simulink library "ControLibrary"  (R2015b)
settings: Solver=ode45  SolverMode=SingleTasking  StartTime=0.0  StopTime=10.0  RelTol=1e-3
values from neighbouring files (symbols this model uses):
  ControlSampleTime = 1/8000    (= 0.000125)    [initTPHardware.m]
  DCCC = initDCCC(LCL,SM)    [Sim_TP3_VSM_init.m]    (also in initDCCC.m = initHSS(LCL,SM))
undefined symbols (not defined in the file or in its folder): CCCTRL, DiscIntNeverNeededParam, VSMCTRL
undefined symbols (not defined in the file): HSS, VSMCC
libraries: FriedrichLibrary x46, simulink x23, simulink_extras x4, ControLibrary x2, ctrl_basic x2
(part 3 of 4)

== system ControLibrary/HSS/CONTROL/i_pi ==
  w : Inport
  x : Inport  Port=2
  umax : Inport  Port=3
  umin : Inport  Port=4
  x0 : Inport  Port=5
  Enable : EnablePort  StatesWhenEnabling=reset
  Discrete-Time Integrator : DiscreteIntegrator  InitialConditionSource=external  InitialConditionSetting=State (most efficient)  SampleTime=ControlSampleTime  ICPrevOutput=DiscIntNeverNeededParam  ICPrevScaledInput=DiscIntNeverNeededParam
  Sum : Sum  Inputs=|+-
  Sum1 : Sum  Inputs=|+-
  Sum2 : Sum  Inputs=++|
  Sum3 : Sum  Inputs=++|
  dynsat : simulink/Discontinuities/Saturation Dynamic  OutMin=[]  OutMax=[]  OutDataTypeStr=Inherit: Same as second input  OutDataType=fixdt(1, 16)  OutScaling=2^-10  DoSatur=off
  kaw : Gain  Gain=ki
  ki : Gain  Gain=ki
  kp : Gain  Gain=kp
  u : Outport
  wires:
  w/1 -> Sum/1
  x/1 -> Sum/2
  Sum/1 -> ki/1, kp/1
  Sum2/1 -> dynsat/2, Sum1/2
  dynsat/1 -> Sum1/1, u/1
  umin/1 -> dynsat/3
  umax/1 -> dynsat/1
  x0/1 -> Discrete-Time Integrator/2
  Discrete-Time Integrator/1 -> Sum2/1
  kp/1 -> Sum2/2
  ki/1 -> Sum3/2
  Sum3/1 -> Discrete-Time Integrator/1
  Sum1/1 -> kaw/1
  kaw/1 -> Sum3/1

== system ControLibrary/HSS/CONTROL/u_pi ==
  w : Inport
  x : Inport  Port=2
  umax : Inport  Port=3
  umin : Inport  Port=4
  x0 : Inport  Port=5
  Enable : EnablePort  StatesWhenEnabling=reset
  Discrete-Time Integrator : DiscreteIntegrator  InitialConditionSource=external  InitialConditionSetting=State (most efficient)  SampleTime=ControlSampleTime  ICPrevOutput=DiscIntNeverNeededParam  ICPrevScaledInput=DiscIntNeverNeededParam
  Sum : Sum  Inputs=|+-
  Sum1 : Sum  Inputs=|+-
  Sum2 : Sum  Inputs=++|
  Sum3 : Sum  Inputs=++|
  dynsat : simulink/Discontinuities/Saturation Dynamic  OutMin=[]  OutMax=[]  OutDataTypeStr=Inherit: Same as second input  OutDataType=fixdt(1, 16)  OutScaling=2^-10  DoSatur=off
  kaw : Gain  Gain=ki
  ki : Gain  Gain=ki
  kp : Gain  Gain=kp
  u : Outport
  wires:
  w/1 -> Sum/1
  x/1 -> Sum/2
  Sum/1 -> ki/1, kp/1
  Sum2/1 -> dynsat/2, Sum1/2
  dynsat/1 -> Sum1/1, u/1
  umin/1 -> dynsat/3
  umax/1 -> dynsat/1
  x0/1 -> Discrete-Time Integrator/2
  Discrete-Time Integrator/1 -> Sum2/1
  kp/1 -> Sum2/2
  ki/1 -> Sum3/2
  Sum3/1 -> Discrete-Time Integrator/1
  Sum1/1 -> kaw/1
  kaw/1 -> Sum3/1

== system ControLibrary/HSS/MANAGEMENT/RateLimit ==
  sp_DCBus : Inport
  ms_dcbus : Inport  Port=2
  Enable : EnablePort  StatesWhenEnabling=reset
  Abs : Abs
  Abs1 : Abs
  Add : Sum  Inputs=+-
  Add1 : Sum  Inputs=+-
  Compare To Constant1 : simulink/Logic and Bit Operations/Compare To Constant  relop=<  const=1  OutDataTypeStr=boolean
  Compare To Constant2 : simulink/Logic and Bit Operations/Compare To Constant  relop=<  const=10  OutDataTypeStr=boolean
  Constant : Constant  Value=UDCbusSpRateUp  SampleTime=ControlSampleTime
  Constant1 : Constant  Value=UDCbusSpRateDown  SampleTime=ControlSampleTime
  Ground : Ground
  Logical Operator : Logic  AllPortsSameDT=off  OutDataTypeStr=boolean
  S-R Flip-Flop : simulink_extras/Flip Flops/S-R Flip-Flop  initial_condition=0
  Saturation Dynamic : simulink/Discontinuities/Saturation Dynamic  OutMin=[]  OutMax=[]  OutDataTypeStr=Inherit: Same as second input  OutDataType=fixdt(1, 16)  OutScaling=2^-10  DoSatur=off
  Terminator : Terminator
  Vdc max : Constant  Value=UDCbusSpMax  SampleTime=ControlSampleTime
  Vdc min : Constant  Value=UDCbusSpMin  SampleTime=ControlSampleTime
  ratelimit1 : Subsystem  mask{Ts=ControlSampleTime}
      mask DialogControl ParameterGroupVar Prompt: Rate Limiter
  sp_DCBus_slow : Outport
  DCBus_isset : Outport  Port=2
  wires:
  ms_dcbus/1 -> ratelimit1/4(x0), Add1/2
  S-R Flip-Flop/1 -> DCBus_isset/1
  Ground/1 -> S-R Flip-Flop/2
  S-R Flip-Flop/2 -> Terminator/1
  Logical Operator/1 -> S-R Flip-Flop/1
  Compare To Constant2/1 -> Logical Operator/2
  Compare To Constant1/1 -> Logical Operator/1
  Abs1/1 -> Compare To Constant2/1
  Add1/1 -> Abs1/1
  Abs/1 -> Compare To Constant1/1
  Add/1 -> Abs/1
  Vdc max/1 -> Saturation Dynamic/1
  sp_DCBus/1 -> Saturation Dynamic/2
  Constant/1 -> ratelimit1/1(rateup)
  Constant1/1 -> ratelimit1/3(ratedown)
  Saturation Dynamic/1 -> ratelimit1/2(x), Add/2
  ratelimit1/1(x_slow) -> sp_DCBus_slow/1, Add/1, Add1/1
  Vdc min/1 -> Saturation Dynamic/3

== system ControLibrary/HSS/Meas/SI -> pu ==
  MeasIn : Inport
  Bus Creator1 : BusCreator  Inputs=5
  Bus Selector : BusSelector  OutputSignals=meas_u_out,meas_i_out,meas_i_inverter,meas_u_dc,meas_u_cap
  Normalize : Gain  Gain=1/PU.Ub  OutDataTypeStr=double  RndMeth=Round
  Normalize1 : Gain  Gain=1/PU.Ib  OutDataTypeStr=double  RndMeth=Round
  Normalize2 : Gain  Gain=1/PU.Ib  OutDataTypeStr=double  RndMeth=Round
  Normalize3 : Gain  Gain=1/PU.Ub  OutDataTypeStr=double  RndMeth=Round
  Normalize4 : Gain  Gain=1/PU.Ub/2  OutDataTypeStr=double  RndMeth=Round
  MeasOut : Outport
  wires:
  MeasIn/1 -> Bus Selector/1
  Normalize/1 -> Bus Creator1/1  "meas_u_out"
  Normalize1/1 -> Bus Creator1/3  "meas_i_inverter"
  Normalize2/1 -> Bus Creator1/2  "meas_i_out"
  Normalize4/1 -> Bus Creator1/4  "meas_vol_dc"
  Bus Creator1/1 -> MeasOut/1
  Bus Selector/1 -> Normalize/1  "<meas_u_out>"
  Bus Selector/2 -> Normalize2/1  "<meas_i_out>"
  Bus Selector/3 -> Normalize1/1  "<meas_i_inverter>"
  Bus Selector/4 -> Normalize4/1  "<meas_u_dc>"
  Bus Selector/5 -> Normalize3/1  "<meas_u_cap>"
  Normalize3/1 -> Bus Creator1/5  "meas_u_cap"

== system ControLibrary/VSM/CONTROL/VSMOC ==
  Manage : Inport
  Meas : Inport  Port=2
  u_inv_dq : Inport  Port=3
  Bus Selector1 : BusSelector  OutputSignals=enable_VSM.enable_ctrl,Param.VSM,enable_VSM.enable_inertia,sp_VSM
  Bus Selector11 : BusSelector  OutputSignals=phi
  Bus Selector2 : BusSelector  OutputSignals=PQ,PLL,u_cap.u_cap_dq0
  Selector : Selector  InputPortWidth=3  IndexOptions=Index vector (dialog)  Indices=[1 2]  OutputSizes=1
  Switch : Switch  Criteria=u2 ~= 0
  VSMOC : Subsystem
  phi_rad : Outport
  sp_u_inv_dq : Outport  Port=2  InitialOutput=[1 0]
  VSMdiag : Outport  Port=3
  wires:
  Selector/1 -> VSMOC/6(u_cap_dq0)
  Bus Selector2/3 -> Selector/1  "<u_cap_dq0>"
  u_inv_dq/1 -> VSMOC/7(u_inv_dq)
  Bus Selector1/4 -> VSMOC/3(sp_VSM)  "<sp_VSM>"
  Bus Selector1/3 -> VSMOC/2(enable_inertia)  "<enable_inertia>"
  Bus Selector1/2 -> VSMOC/1(Param)  "<VSM>"
  Bus Selector2/2 -> Bus Selector11/1, VSMOC/5(PLL)  "<PLL>"
  Bus Selector2/1 -> VSMOC/4(PQ_meas)  "<PQ>"
  Meas/1 -> Bus Selector2/1
  Bus Selector1/1 -> Switch/2, VSMOC/Enable  "<enable_ctrl>"
  Manage/1 -> Bus Selector1/1
  Switch/1 -> phi_rad/1
  VSMOC/2(sp_u_inv_dq) -> sp_u_inv_dq/1
  VSMOC/3(VSMdiag) -> VSMdiag/1
  VSMOC/1(phi_rad) -> Switch/1
  Bus Selector11/1 -> Switch/3  "<phi>"

== system ControLibrary/VSM/CONTROL/active_damping ==
  enable_damp_dq : Inport
  Reset : Inport  Port=2
  u_dq0 : Inport  Port=3
  Phi : Inport  Port=4
  Bus Selector : BusSelector  OutputSignals=Damp_dq,Damp_dq,Damp_CM,OmLead,OmLag
  Integrator (inertia) : DiscreteIntegrator  gainval=1  ExternalReset=rising  InitialConditionSource=external  InitialCondition=1  InitialConditionSetting=State (most efficient)  SampleTime=ControlSampleTime  ICPrevOutput=DiscIntNeverNeededParam  ICPrevScaledInput=DiscIntNeverNeededParam
  Mux : Mux  Inputs=3
  Product{,1..3} (4 alike) : Product
  Sum : Sum  Inputs=|+-
  Sum2 : Sum  Inputs=++|
  Unit Delay2 : UnitDelay  InitialCondition=[0 0 0]  SampleTime=ControlSampleTime
  dq0->ab0 phi : FriedrichLibrary/Transformations/dq0->ab0 phi  SystemSampleTime=-1
  damp_dq0 : Outport
  wires:
  Bus Selector/5 -> Product3/2  "<OmLag>"
  Bus Selector/4 -> Product2/1  "<OmLead>"
  dq0->ab0 phi/1 -> Integrator (inertia)/3
  Unit Delay2/1 -> dq0->ab0 phi/1
  Reset/1 -> Integrator (inertia)/2
  Phi/1 -> dq0->ab0 phi/2
  Product1/1 -> damp_dq0/1
  Mux/1 -> Product/1, Product1/1  "enable"
  Product/1 -> Product2/2, Sum2/1
  u_dq0/1 -> Product/2
  Bus Selector/3 -> Mux/3  "<Damp_CM>"
  Bus Selector/2 -> Mux/2  "<Damp_dq>"
  Bus Selector/1 -> Mux/1  "<Damp_dq>"
  enable_damp_dq/1 -> Bus Selector/1
  Sum/1 -> Integrator (inertia)/1
  Sum2/1 -> Product1/2, Product3/1
  Product3/1 -> Sum/2
  Integrator (inertia)/1 -> Sum2/2, Unit Delay2/1
  Product2/1 -> Sum/1

== system ControLibrary/VSM/CONTROL/dq0 to duty ==
  phi_rad : Inport
  u_dq0 : Inport  Port=2
  u_dc : Inport  Port=3
  Bias : Bias  Bias=Ctrl.PWM.tauT*Ctrl.PU.omegab
  Bus Creator3 : BusCreator  Inputs=2
  Divide : Product  Inputs=*/
  Gain : Gain  Gain=eye(NrChannels,3)  Multiplication=Matrix(K*u)
  Modulation : FriedrichLibrary/Transformations/Modulation  Method=Sine Modulation  Ts=ControlSampleTime
  Saturation : Saturate  UpperLimit=inf  LowerLimit=1
  Signal Specification1 : SignalSpecification
  dq0->ab0 phi : FriedrichLibrary/Transformations/dq0->ab0 phi  SystemSampleTime=-1
  d : Outport
  pwmDiag : Outport  Port=2
  wires:
  Signal Specification1/1 -> d/1
  Gain/1 -> Signal Specification1/1, Bus Creator3/1  "pwm"
  Bus Creator3/1 -> pwmDiag/1  "pwmDiag"
  Saturation/1 -> Divide/2
  u_dc/1 -> Saturation/1
  Bias/1 -> dq0->ab0 phi/2
  Modulation/1 -> Gain/1
  dq0->ab0 phi/1 -> Divide/1
  Divide/1 -> Modulation/1  "ab0 norm"
  u_dq0/1 -> dq0->ab0 phi/1
  phi_rad/1 -> Bias/1, Bus Creator3/2  "phi"

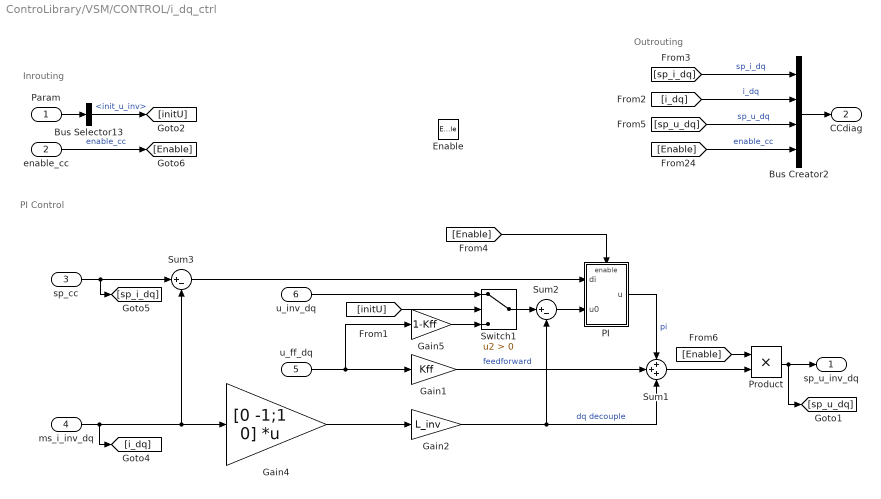
== system ControLibrary/VSM/CONTROL/i_dq_ctrl ==
  note: PI Control
  note: Outrouting
  note: Inrouting
  Param : Inport
  enable_cc : Inport  Port=2
  sp_cc : Inport  Port=3
  ms_i_inv_dq : Inport  Port=4
  u_ff_dq : Inport  Port=5
  u_inv_dq : Inport  Port=6
  Enable : EnablePort  StatesWhenEnabling=reset
  Bus Creator2 : BusCreator  Inputs=4
  Bus Selector13 : BusSelector  OutputSignals=init_u_inv
  Gain1 : Gain  Gain=Kff
  Gain2 : Gain  Gain=L_inv
  Gain4 : Gain  Gain=[0 -1;1 0]  Multiplication=Matrix(K*u)
  Gain5 : Gain  Gain=1-Kff
  PI : Subsystem
  Product : Product
  Sum1 : Sum  Inputs=+++
  Sum2 : Sum  Inputs=|+-
  Sum3 : Sum  Inputs=|+-
  Switch1 : Switch  Criteria=u2 > Threshold
  sp_u_inv_dq : Outport
  CCdiag : Outport  Port=2
  wires:
  Gain5/1 -> Switch1/3
  u_ff_dq/1 -> Gain5/1, Gain1/1
  [i_dq] -> Bus Creator2/2  "i_dq"
  [sp_i_dq] -> Bus Creator2/1  "sp_i_dq"
  Bus Creator2/1 -> CCdiag/1
  [Enable] -> Bus Creator2/4  "enable_cc"
  enable_cc/1 -> [Enable]  "enable_cc"
  [sp_u_dq] -> Bus Creator2/3  "sp_u_dq"
  Product/1 -> [sp_u_dq], sp_u_inv_dq/1
  [Enable] -> Product/1
  Bus Selector13/1 -> [initU]  "<init_u_inv>"
  Param/1 -> Bus Selector13/1
  sp_cc/1 -> [sp_i_dq], Sum3/1
  ms_i_inv_dq/1 -> Gain4/1, Sum3/2, [i_dq]
  Sum3/1 -> PI/1(di)
  [Enable] -> PI/Enable
  PI/1(u) -> Sum1/1  "pi"
  u_inv_dq/1 -> Switch1/1
  Sum1/1 -> Product/2
  [initU] -> Switch1/2
  Gain2/1 -> Sum2/2, Sum1/3  "dq decouple"
  Gain1/1 -> Sum1/2  "feedforward"
  Gain4/1 -> Gain2/1
  Sum2/1 -> PI/2(u0)
  Switch1/1 -> Sum2/1

== system ControLibrary/VSM/CONTROL/re_init ==
  Uset : Inport
  Uvr : Inport  Port=2
  Trigger : TriggerPort  PortDimensions=1
  MATLAB Function : MATLAB Function  TreatAsAtomicUnit=on
  Terminator : Terminator
  Uinit : Outport
  Phi : Outport  Port=2
  wires:
  MATLAB Function/2(Phi) -> Phi/1
  Uvr/1 -> MATLAB Function/2(Uvr)
  Uset/1 -> MATLAB Function/1(Uset)
  MATLAB Function/1(Uinit) -> Uinit/1
  MATLAB Function/3(UvrShift) -> Terminator/1

== system ControLibrary/VSM/MANAGEMENT/current_watchdog ==
  |i| set : Inport
  |i| reset : Inport  Port=2
  i_ab : Inport  Port=3
  sp_gain : Inport  Port=4
  active_current_watchdog : EnablePort  StatesWhenEnabling=reset
  Divide : Product  Inputs=/**
  Math Function1 : Math  Operator=square  SaturateOnIntegerOverflow=on
  Math Function2 : Math  Operator=square  SaturateOnIntegerOverflow=on
  Math Function3 : Math  Operator=square  SaturateOnIntegerOverflow=on
  Relational Operator : RelationalOperator  Operator=<=  OutDataTypeStr=boolean
  Relational Operator1 : RelationalOperator  Operator=<=  OutDataTypeStr=boolean
  S-R Flip-Flop1 : simulink_extras/Flip Flops/S-R Flip-Flop  initial_condition=0
  Sum of Elements1 : Sum  Inputs=+
  Terminator1 : Terminator
  enable_cc : Outport
  sp_gain_wd : Outport  Port=2
  wires:
  Divide/1 -> sp_gain_wd/1
  sp_gain/1 -> Divide/3
  |i| set/1 -> Math Function2/1, Divide/1
  |i| reset/1 -> Math Function3/1, Divide/2
  Math Function3/1 -> Relational Operator1/2
  S-R Flip-Flop1/1 -> enable_cc/1
  S-R Flip-Flop1/2 -> Terminator1/1
  Relational Operator/1 -> S-R Flip-Flop1/1
  Relational Operator1/1 -> S-R Flip-Flop1/2
  Math Function1/1 -> Sum of Elements1/1
  Sum of Elements1/1 -> Relational Operator/2, Relational Operator1/1
  i_ab/1 -> Math Function1/1
  Math Function2/1 -> Relational Operator/1

== system ControLibrary/VSM/MANAGEMENT/i_sp_dq_generator ==
  sp_gain : Inport
  i_dq : Inport  Port=2
  Trigger : TriggerPort  PortDimensions=1
  Gain : Gain  Commented=on  Gain=0.95/1.5
  Gain1 : Gain  Commented=on  Gain=eye(2,1)
  Gain3 : Gain  Commented=on  Gain=0.5
  Math Function : Math  Commented=on  Operator=square  SaturateOnIntegerOverflow=on
  Product : Product
  Saturation : Saturate  UpperLimit=1  LowerLimit=-1
  Saturation1 : Saturate  UpperLimit=1  LowerLimit=-1
  Sqrt : Sqrt  Commented=on  SaturateOnIntegerOverflow=on
  Sum of Elements : Sum  Commented=on  Inputs=+
  Terminator : Terminator  Commented=on
  Terminator1 : Terminator  Commented=on
  i_dq_spt : Outport
  wires:
  Saturation/1 -> Product/1
  sp_gain/1 -> Saturation/1
  Gain3/1 -> Terminator1/1
  Gain/1 -> Terminator/1
  i_dq/1 -> Product/2, Gain/1, Math Function/1
  Math Function/1 -> Sum of Elements/1
  Sum of Elements/1 -> Sqrt/1
  Sqrt/1 -> Gain1/1
  Gain1/1 -> Gain3/1
  Product/1 -> Saturation1/1
  Saturation1/1 -> i_dq_spt/1

== system ControLibrary/VSM/MANAGEMENT/sp_VSM ==
  EnableRateLimit : Inport
  CMD : Inport  Port=2
  MEAS : Inport  Port=3
  Bus Creator : BusCreator  Inputs=3
  Bus Selector1 : BusSelector  OutputSignals=u_out.u_out_ab0
  Bus Selector6 : BusSelector  OutputSignals=Param.VSM.sp_f,Param.VSM.sp_E,Param.VSM.sp_PQ,Param.VSM.sp_PQ_limit
  "CMD " : InportShadow  Port=2
  E(PQ) : Subsystem
  PQ(U) Limit : Subsystem
  RateLimit : Subsystem
  Saturation : Saturate  UpperLimit=1  LowerLimit=-1
  sp_VSM : Outport
  wires:
  Saturation/1 -> RateLimit/1(PQ)
  "CMD "/1 -> E(PQ)/2(cmd)
  Bus Creator/1 -> sp_VSM/1
  Bus Selector6/1 -> Bus Creator/1  "<sp_f>"
  MEAS/1 -> Bus Selector1/1
  CMD/1 -> Bus Selector6/1
  PQ(U) Limit/1(sp_PQ_limit) -> Bus Creator/3  "sp_PQ"
  Bus Selector6/4 -> PQ(U) Limit/2(enable)  "<sp_PQ_limit>"
  Bus Selector1/1 -> PQ(U) Limit/3(u_out)  "<u_out_ab0>"
  RateLimit/1(PQslow) -> PQ(U) Limit/1(sp_PQ), E(PQ)/3(sp_PQ)
  EnableRateLimit/1 -> RateLimit/Enable  "ENABLED"
  Bus Selector6/3 -> Saturation/1  "<sp_PQ>"
  Bus Selector6/2 -> E(PQ)/1(E)  "<sp_E>"
  E(PQ)/1(sp_E) -> Bus Creator/2  "sp_E"

== system ControLibrary/VSM/Meas/SI -> pu ==
  MeasIn : Inport
  Bus Creator1 : BusCreator  Inputs=5
  Bus Selector : BusSelector  OutputSignals=meas_u_out,meas_i_out,meas_i_inverter,meas_u_dc,meas_u_cap
  Normalize : Gain  Gain=1/PU.Ub  OutDataTypeStr=double  RndMeth=Round
  Normalize1 : Gain  Gain=1/PU.Ib  OutDataTypeStr=double  RndMeth=Round
  Normalize2 : Gain  Gain=1/PU.Ib  OutDataTypeStr=double  RndMeth=Round
  Normalize3 : Gain  Gain=1/PU.Ub  OutDataTypeStr=double  RndMeth=Round
  Normalize4 : Gain  Gain=1/PU.Ub/2  OutDataTypeStr=double  RndMeth=Round
  MeasOut : Outport
  wires:
  MeasIn/1 -> Bus Selector/1
  Normalize/1 -> Bus Creator1/1  "meas_u_out"
  Normalize1/1 -> Bus Creator1/3  "meas_i_inverter"
  Normalize2/1 -> Bus Creator1/2  "meas_i_out"
  Normalize4/1 -> Bus Creator1/4  "meas_vol_dc"
  Bus Creator1/1 -> MeasOut/1
  Bus Selector/1 -> Normalize/1  "<meas_u_out>"
  Bus Selector/2 -> Normalize2/1  "<meas_i_out>"
  Bus Selector/3 -> Normalize1/1  "<meas_i_inverter>"
  Bus Selector/4 -> Normalize4/1  "<meas_u_dc>"
  Bus Selector/5 -> Normalize3/1  "<meas_u_cap>"
  Normalize3/1 -> Bus Creator1/5  "meas_u_cap"

== system ControLibrary/VSM/Meas/meas_i_inv ==
  abc : Inport
  phi : Inport  Port=2
  Bus Creator1 : BusCreator  Inputs=3
  PhN->ab2 : FriedrichLibrary/Transformations/PhN->ab0  SystemSampleTime=-1
  ab0->dq0-faster : FriedrichLibrary/Transformations/ab0->dq0-faster  SystemSampleTime=-1
  i_inv_x : Outport
  wires:
  Bus Creator1/1 -> i_inv_x/1
  phi/1 -> ab0->dq0-faster/2
  abc/1 -> PhN->ab2/1, Bus Creator1/1  "i_inv_abc"
  PhN->ab2/1 -> ab0->dq0-faster/1, Bus Creator1/2  "i_inv_ab0"
  ab0->dq0-faster/1 -> Bus Creator1/3  "i_inv_dq0"

== system ControLibrary/VSM/Meas/meas_i_out ==
  abc : Inport
  phi : Inport  Port=2
  Bus Creator1 : BusCreator  Inputs=3
  PhN->ab2 : FriedrichLibrary/Transformations/PhN->ab0  SystemSampleTime=-1
  ab0->dq0-faster : FriedrichLibrary/Transformations/ab0->dq0-faster  SystemSampleTime=-1
  i_out_x : Outport
  wires:
  Bus Creator1/1 -> i_out_x/1
  phi/1 -> ab0->dq0-faster/2
  abc/1 -> PhN->ab2/1, Bus Creator1/1  "i_out_abc"
  PhN->ab2/1 -> ab0->dq0-faster/1, Bus Creator1/2  "i_out_ab0"
  ab0->dq0-faster/1 -> Bus Creator1/3  "i_out_dq0"

== system ControLibrary/VSM/Meas/meas_u_cap ==
  abc : Inport
  phi : Inport  Port=2
  Bus Creator1 : BusCreator  Inputs=3
  PhN->ab2 : FriedrichLibrary/Transformations/PhN->ab0  SystemSampleTime=-1
  ab0->dq0-faster : FriedrichLibrary/Transformations/ab0->dq0-faster  SystemSampleTime=-1
  u_cap_x : Outport
  wires:
  ab0->dq0-faster/1 -> Bus Creator1/3  "u_cap_dq0"
  PhN->ab2/1 -> Bus Creator1/2, ab0->dq0-faster/1  "u_cap_ab0"
  abc/1 -> Bus Creator1/1, PhN->ab2/1  "u_cap_abc"
  phi/1 -> ab0->dq0-faster/2
  Bus Creator1/1 -> u_cap_x/1

== system ControLibrary/VSM/Meas/meas_u_out ==
  abc : Inport
  phi : Inport  Port=2
  Bus Creator1 : BusCreator  Inputs=3
  PhN->ab2 : FriedrichLibrary/Transformations/PhN->ab0  SystemSampleTime=-1
  ab0->dq0-faster : FriedrichLibrary/Transformations/ab0->dq0-faster  SystemSampleTime=-1
  u_out_x : Outport
  wires:
  ab0->dq0-faster/1 -> Bus Creator1/3  "u_out_dq0"
  PhN->ab2/1 -> Bus Creator1/2, ab0->dq0-faster/1  "u_out_ab0"
  abc/1 -> Bus Creator1/1, PhN->ab2/1  "u_out_abc"
  phi/1 -> ab0->dq0-faster/2
  Bus Creator1/1 -> u_out_x/1

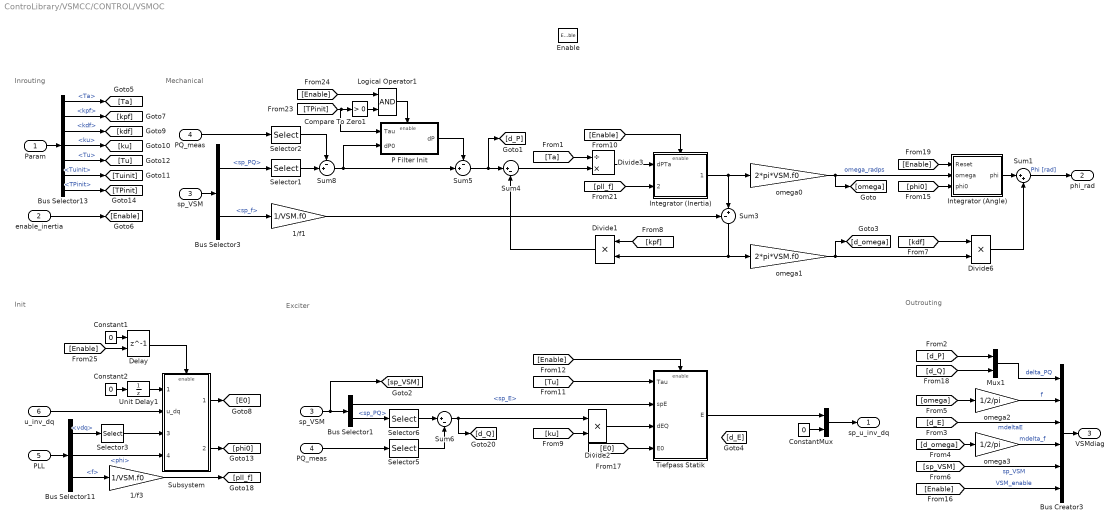
== system ControLibrary/VSMCC/CONTROL/VSMOC ==
  note: Inrouting
  note: Mechanical
  note: Exciter
  note: Init
  note: Outrouting
  Param : Inport
  enable_inertia : Inport  Port=2
  sp_VSM : Inport  Port=3
  PQ_meas : Inport  Port=4
  PLL : Inport  Port=5
  u_inv_dq : Inport  Port=6
  Enable : EnablePort  StatesWhenEnabling=reset
  1/f1 : Gain  Gain=1/VSM.f0
  1/f3 : Gain  Gain=1/VSM.f0
  Bus Creator3 : BusCreator  Inputs=6
  Bus Selector1 : BusSelector  OutputSignals=sp_E,sp_PQ
  Bus Selector11 : BusSelector  OutputSignals=vdq,phi,f
  Bus Selector13 : BusSelector  OutputSignals=Ta,kpf,kdf,ku,Tu,Tuinit,TPinit
  Bus Selector3 : BusSelector  OutputSignals=sp_PQ,sp_f
  Compare To Zero1 : simulink/Logic and Bit Operations/Compare To Zero  relop=>  OutDataTypeStr=boolean
  Constant : Constant  Value=0
  Constant1 : Constant  Value=0  SampleTime=ControlSampleTime
  Constant2 : Constant  Value=0  SampleTime=ControlSampleTime
  Delay : Delay  DelayLength=1  InitialCondition=1  ExternalReset=Rising
      settings: InputPortMap=u0,r5
  Divide1 : Product  Inputs=**
  Divide2 : Product  Inputs=**
  Divide3 : Product  Inputs=/*
  Divide6 : Product  Inputs=**
  Integrator (Angle) : Subsystem
  Integrator (Inertia) : Subsystem
  Logical Operator1 : Logic  AllPortsSameDT=off  OutDataTypeStr=boolean
  Mux : Mux  Inputs=2
  Mux1 : Mux  Inputs=2
  P Filter Init : Subsystem
  "PQ_meas " : InportShadow  Port=4
  Selector1 : Selector  InputPortWidth=2  IndexOptions=Index vector (dialog)  Indices=1  OutputSizes=1
  Selector2 : Selector  InputPortWidth=2  IndexOptions=Index vector (dialog)  Indices=1  OutputSizes=1
  Selector3 : Selector  InputPortWidth=3  IndexOptions=Index vector (dialog)  Indices=[1 2]  OutputSizes=1
  Selector5 : Selector  InputPortWidth=2  IndexOptions=Index vector (dialog)  Indices=2  OutputSizes=1
  Selector6 : Selector  InputPortWidth=2  IndexOptions=Index vector (dialog)  Indices=2  OutputSizes=1
  Subsystem : Subsystem
  Sum1 : Sum  Inputs=|++
  Sum3 : Sum  Inputs=-+|
  Sum4 : Sum  Inputs=|+-
  Sum5 : Sum  Inputs=-+|
  Sum6 : Sum  Inputs=|+-
  Sum8 : Sum  Inputs=-+|
  Tiefpass Statik : Subsystem
  Unit Delay1 : UnitDelay  InitialCondition=1  SampleTime=ControlSampleTime
  omega0 : Gain  Gain=2*pi*VSM.f0
  omega1 : Gain  Gain=2*pi*VSM.f0
  omega2 : Gain  Gain=1/2/pi
  omega3 : Gain  Gain=1/2/pi
  "sp_VSM " : InportShadow  Port=3
  sp_u_inv_dq : Outport  InitialOutput=[1 0]
  phi_rad : Outport  Port=2
  VSMdiag : Outport  Port=3
  wires:
  Tiefpass Statik/1(E) -> Mux/1
  Divide6/1 -> Sum1/2
  Bus Selector11/2 -> Subsystem/4(phi_pll)  "<phi>"
  Bus Selector1/1 -> Tiefpass Statik/2(spE)  "<sp_E>"
  Selector5/1 -> Sum6/2
  Selector6/1 -> Sum6/1
  1/f1/1 -> Sum3/1
  [d_Q] -> Mux1/2
  [d_P] -> Mux1/1
  Mux1/1 -> Bus Creator3/1  "delta_PQ"
  Selector2/1 -> Sum8/1
  Sum6/1 -> [d_Q], Divide2/1
  "sp_VSM "/1 -> Bus Selector1/1, [sp_VSM]
  Bus Selector1/2 -> Selector6/1  "<sp_PQ>"
  "PQ_meas "/1 -> Selector5/1
  sp_VSM/1 -> Bus Selector3/1
  [phi0] -> Integrator (Angle)/3(phi0)
  [kpf] -> Divide1/1
  [kdf] -> Divide6/1
  1/f3/1 -> [pll_f]
  Bus Selector11/3 -> 1/f3/1  "<f>"
  Integrator (Angle)/1(phi) -> Sum1/1
  Selector3/1 -> Subsystem/3(u_dq_pll)
  Divide2/1 -> Tiefpass Statik/3(dEQ)
  ? -> [d_E]
  [Enable] -> Tiefpass Statik/Enable
  [Tu] -> Tiefpass Statik/1(Tau)
  [Enable] -> Bus Creator3/6  "VSM_enable"
  [ku] -> Divide2/2
  [Ta] -> Divide3/1
  [Enable] -> Integrator (Inertia)/Enable
  Sum1/1 -> phi_rad/1  "Phi [rad]"
  Divide1/1 -> Sum4/2
  Sum4/1 -> Divide3/2
  Sum3/1 -> omega1/1, Divide1/2
  omega0/1 -> [omega], Integrator (Angle)/2(omega)  "omega_radps"
  Bus Selector3/1 -> Selector1/1  "<sp_PQ>"
  Bus Selector3/2 -> 1/f1/1  "<sp_f>"
  PLL/1 -> Bus Selector11/1
  Bus Creator3/1 -> VSMdiag/1
  [omega] -> omega2/1
  omega1/1 -> [d_omega], Divide6/2
  [d_E] -> Bus Creator3/3  "mdeltaE"
  [d_omega] -> omega3/1
  omega2/1 -> Bus Creator3/2  "f"
  omega3/1 -> Bus Creator3/4  "mdelta_f"
  [sp_VSM] -> Bus Creator3/5  "sp_VSM"
  PQ_meas/1 -> Selector2/1
  Bus Selector11/1 -> Selector3/1  "<vdq>"
  Integrator (Inertia)/1(omega) -> omega0/1, Sum3/2
  Divide3/1 -> Integrator (Inertia)/1(dPTa)
  [pll_f] -> Integrator (Inertia)/2(omega_0)
  Mux/1 -> sp_u_inv_dq/1
  Constant/1 -> Mux/2
  Subsystem/1(u_abs) -> [E0]
  Subsystem/2(u_ang) -> [phi0]
  [Enable] -> Integrator (Angle)/1(Reset)
  [E0] -> Tiefpass Statik/4(E0)
  Constant1/1 -> Delay/1
  Delay/1 -> Subsystem/Enable
  Selector1/1 -> Sum8/2
  Sum5/1 -> Sum4/1, [d_P]
  Sum8/1 -> Sum5/2, P Filter Init/2(dP0)
  [TPinit] -> P Filter Init/1(Tau), Compare To Zero1/1
  P Filter Init/1(dP) -> Sum5/1
  Compare To Zero1/1 -> Logical Operator1/2
  Logical Operator1/1 -> P Filter Init/Enable
  [Enable] -> Logical Operator1/1
  Bus Selector13/6 -> [Tuinit]  "<Tuinit>"
  Bus Selector13/5 -> [Tu]  "<Tu>"
  Bus Selector13/4 -> [ku]  "<ku>"
  Bus Selector13/3 -> [kdf]  "<kdf>"
  Bus Selector13/2 -> [kpf]  "<kpf>"
  Bus Selector13/1 -> [Ta]  "<Ta>"
  Param/1 -> Bus Selector13/1
  Bus Selector13/7 -> [TPinit]  "<TPinit>"
  enable_inertia/1 -> [Enable]
  [Enable] -> Delay/2
  u_inv_dq/1 -> Subsystem/2(u_dq)
  Constant2/1 -> Unit Delay1/1
  Unit Delay1/1 -> Subsystem/1(first_run)

== system ControLibrary/VSMCC/CONTROL/active_damping ==
  enable_damp_dq : Inport
  enable_damp_cm : Inport  Port=2
  u_dq0 : Inport  Port=3
  Mux : Mux  Inputs=2
  Selector : Selector  InputPortWidth=3  IndexOptions=Index vector (dialog)  Indices=[3]  OutputSizes=1
  Selector1 : Selector  InputPortWidth=3  IndexOptions=Index vector (dialog)  Indices=[1 2]  OutputSizes=1
  VTFF - HighPass1 : Subsystem  mask{Gain=Ctrl.VTFF.Gain, Tlead=Ctrl.VTFF.Tlead, Tlag=Ctrl.VTFF.Tlag}
      mask init:
      | if Tlag==0
      |     OmLag=0;
      | else
      |     OmLag=1/Tlag;
      | end
      mask DialogControl ParameterGroupVar Prompt: Lead Lag Filter
  VTFF - HighPass2 : Subsystem  mask{Gain=Ctrl.VTFF.Gain, Tlead=Ctrl.VTFF.Tlead, Tlag=Ctrl.VTFF.Tlag}
      mask init:
      | if Tlag==0
      |     OmLag=0;
      | else
      |     OmLag=1/Tlag;
      | end
      mask DialogControl ParameterGroupVar Prompt: Lead Lag Filter
  damp_dq0 : Outport
  wires:
  u_dq0/1 -> Selector1/1, Selector/1
  Selector/1 -> VTFF - HighPass1/1(u)
  VTFF - HighPass1/1(x) -> Mux/2  "damp_cm"
  Selector1/1 -> VTFF - HighPass2/1(u)
  VTFF - HighPass2/1(x) -> Mux/1  "damp_dq"
  enable_damp_dq/1 -> VTFF - HighPass2/Enable
  enable_damp_cm/1 -> VTFF - HighPass1/Enable
  Mux/1 -> damp_dq0/1

== system ControLibrary/VSMCC/CONTROL/dq0 to duty ==
  u_dq0 : Inport
  phi_rad : Inport  Port=2
  u_dc : Inport  Port=3
  Bias : Bias  Bias=Ctrl.PWM.tauT*Ctrl.pu.omegab
  Bus Creator3 : BusCreator  Inputs=1
  Divide : Product  Inputs=*/
  Gain : Gain  Gain=eye(NrChannels,3)  Multiplication=Matrix(K*u)
  Modulation : FriedrichLibrary/Transformations/Modulation  Method=Sine Modulation  Ts=ControlSampleTime
  Saturation : Saturate  UpperLimit=inf  LowerLimit=1
  Signal Specification1 : SignalSpecification
  dq0->ab0 phi : FriedrichLibrary/Transformations/dq0->ab0 phi  SystemSampleTime=-1
  d : Outport
  pwmDiag : Outport  Port=2
  wires:
  phi_rad/1 -> Bias/1
  u_dq0/1 -> dq0->ab0 phi/1
  Divide/1 -> Modulation/1  "ab0 norm"
  dq0->ab0 phi/1 -> Divide/1
  Modulation/1 -> Gain/1
  Bias/1 -> dq0->ab0 phi/2
  u_dc/1 -> Saturation/1
  Saturation/1 -> Divide/2
  Bus Creator3/1 -> pwmDiag/1  "pwmDiag"
  Gain/1 -> Bus Creator3/1, Signal Specification1/1  "pwm"
  Signal Specification1/1 -> d/1

== system ControLibrary/VSMCC/CONTROL/i_dq_ctrl ==
  note: PI Control
  note: Outrouting
  note: Inrouting
  Param : Inport
  enable_cc : Inport  Port=2
  sp_cc : Inport  Port=3
  ms_i_inv_dq : Inport  Port=4
  u_ff_dq : Inport  Port=5
  u_inv_dq : Inport  Port=6
  Enable : EnablePort  StatesWhenEnabling=reset
  Bus Creator2 : BusCreator  Inputs=4
  Bus Selector13 : BusSelector  OutputSignals=init_u_inv
  Gain1 : Gain  Gain=Kff
  Gain2 : Gain  Gain=L_inv
  Gain3 : Gain  Gain=1-Kff
  Gain4 : Gain  Gain=[0 -1;1 0]  Multiplication=Matrix(K*u)
  PI : Subsystem
  Product : Product
  Sum1 : Sum  Inputs=+++
  Sum2 : Sum  Inputs=|+-
  Sum3 : Sum  Inputs=|+-
  Switch1 : Switch  Criteria=u2 > Threshold
  sp_u_inv_dq : Outport
  CCdiag : Outport  Port=2
  wires:
  u_ff_dq/1 -> Switch1/3, Gain1/1
  [i_dq] -> Bus Creator2/2  "i_dq"
  [sp_i_dq] -> Bus Creator2/1  "sp_i_dq"
  Bus Creator2/1 -> CCdiag/1
  [Enable] -> Bus Creator2/4  "enable_cc"
  enable_cc/1 -> [Enable]  "enable_cc"
  [sp_u_dq] -> Bus Creator2/3  "sp_u_dq"
  Product/1 -> [sp_u_dq], sp_u_inv_dq/1
  [Enable] -> Product/1
  Bus Selector13/1 -> [initU]  "<init_u_inv>"
  Param/1 -> Bus Selector13/1
  sp_cc/1 -> [sp_i_dq], Sum3/1
  ms_i_inv_dq/1 -> Gain4/1, Sum3/2, [i_dq]
  Sum3/1 -> PI/1(di)
  [Enable] -> PI/Enable
  PI/1(u) -> Sum1/1  "pi"
  u_inv_dq/1 -> Switch1/1
  Sum1/1 -> Product/2
  [initU] -> Switch1/2
  Gain2/1 -> Sum2/2, Sum1/3  "dq decouple"
  Gain1/1 -> Sum1/2  "feedforward"
  Gain4/1 -> Gain2/1
  Sum2/1 -> PI/2(u0)
  Switch1/1 -> Gain3/1
  Gain3/1 -> Sum2/1

== system ControLibrary/VSMCC/MANAGEMENT/current_watchdog ==
  |i| set : Inport
  |i| reset : Inport  Port=2
  i_ab : Inport  Port=3
  sp_gain : Inport  Port=4
  active_current_watchdog : EnablePort  StatesWhenEnabling=reset
  Divide : Product  Inputs=/**
  Math Function1 : Math  Operator=square  SaturateOnIntegerOverflow=on
  Math Function2 : Math  Operator=square  SaturateOnIntegerOverflow=on
  Math Function3 : Math  Operator=square  SaturateOnIntegerOverflow=on
  Relational Operator : RelationalOperator  Operator=<=  OutDataTypeStr=boolean
  Relational Operator1 : RelationalOperator  Operator=<=  OutDataTypeStr=boolean
  S-R Flip-Flop1 : simulink_extras/Flip Flops/S-R Flip-Flop  initial_condition=0
  Sum of Elements1 : Sum  Inputs=+
  Terminator1 : Terminator
  enable_cc : Outport
  sp_gain_wd : Outport  Port=2
  wires:
  i_ab/1 -> Math Function1/1
  Sum of Elements1/1 -> Relational Operator1/1, Relational Operator/2
  Math Function1/1 -> Sum of Elements1/1
  Relational Operator1/1 -> S-R Flip-Flop1/2
  Relational Operator/1 -> S-R Flip-Flop1/1
  S-R Flip-Flop1/2 -> Terminator1/1
  S-R Flip-Flop1/1 -> enable_cc/1
  Math Function2/1 -> Relational Operator/1
  Math Function3/1 -> Relational Operator1/2
  |i| reset/1 -> Divide/2, Math Function3/1
  |i| set/1 -> Divide/1, Math Function2/1
  sp_gain/1 -> Divide/3
  Divide/1 -> sp_gain_wd/1

== system ControLibrary/VSMCC/MANAGEMENT/i_sp_dq_generator ==
  sp_gain : Inport
  i_dq : Inport  Port=2
  Trigger : TriggerPort  PortDimensions=1
  Gain : Gain  Commented=on  Gain=0.95/1.5
  Gain1 : Gain  Commented=on  Gain=eye(2,1)
  Gain3 : Gain  Commented=on  Gain=0.5
  Math Function : Math  Commented=on  Operator=square  SaturateOnIntegerOverflow=on
  Product : Product
  Saturation : Saturate  UpperLimit=1  LowerLimit=-1
  Saturation1 : Saturate  UpperLimit=1  LowerLimit=-1
  Sqrt : Sqrt  Commented=on  SaturateOnIntegerOverflow=on
  Sum of Elements : Sum  Commented=on  Inputs=+
  Terminator : Terminator  Commented=on
  Terminator1 : Terminator  Commented=on
  i_dq_spt : Outport
  wires:
  Product/1 -> Saturation1/1
  Gain1/1 -> Gain3/1
  Sqrt/1 -> Gain1/1
  Sum of Elements/1 -> Sqrt/1
  Math Function/1 -> Sum of Elements/1
  i_dq/1 -> Math Function/1, Gain/1, Product/2
  Gain/1 -> Terminator/1
  Gain3/1 -> Terminator1/1
  sp_gain/1 -> Saturation/1
  Saturation/1 -> Product/1
  Saturation1/1 -> i_dq_spt/1

== system ControLibrary/VSMCC/Meas/SI -> pu ==
  MeasIn : Inport
  Bus Creator1 : BusCreator  Inputs=5
  Bus Selector : BusSelector  OutputSignals=meas_u_out,meas_i_out,meas_i_inverter,meas_u_dc,meas_u_cap
  Normalize : Gain  Gain=1/PU.Vb  OutDataTypeStr=double  RndMeth=Round
  Normalize1 : Gain  Gain=1/PU.Ib  OutDataTypeStr=double  RndMeth=Round
  Normalize2 : Gain  Gain=1/PU.Ib  OutDataTypeStr=double  RndMeth=Round
  Normalize3 : Gain  Gain=1/PU.Vb  OutDataTypeStr=double  RndMeth=Round
  Normalize4 : Gain  Gain=1/PU.Vb/2  OutDataTypeStr=double  RndMeth=Round
  MeasOut : Outport
  wires:
  Normalize3/1 -> Bus Creator1/5  "meas_u_cap"
  Bus Selector/5 -> Normalize3/1  "<meas_u_cap>"
  Bus Selector/4 -> Normalize4/1  "<meas_u_dc>"
  Bus Selector/3 -> Normalize1/1  "<meas_i_inverter>"
  Bus Selector/2 -> Normalize2/1  "<meas_i_out>"
  Bus Selector/1 -> Normalize/1  "<meas_u_out>"
  Bus Creator1/1 -> MeasOut/1
  Normalize4/1 -> Bus Creator1/4  "meas_vol_dc"
  Normalize2/1 -> Bus Creator1/2  "meas_i_out"
  Normalize1/1 -> Bus Creator1/3  "meas_i_inverter"
  Normalize/1 -> Bus Creator1/1  "meas_u_out"
  MeasIn/1 -> Bus Selector/1

== system ControLibrary/DCCC/MANAGEMENT/RateLimit/ratelimit ==
  rateup : Inport
  x : Inport  Port=2
  ratedown : Inport  Port=3
  x0 : Inport  Port=4
  Delay : Delay  DelayLength=1  InitialConditionSource=Input port  SampleTime=Ts
      settings: InputPortMap=u0,p4
  Gain : Gain  Gain=Ts
  Gain1 : Gain  Gain=-Ts
  Saturation Dynamic2 : simulink/Discontinuities/Saturation Dynamic  OutMin=[]  OutMax=[]  OutDataTypeStr=Inherit: Same as second input  OutDataType=fixdt(1, 16)  OutScaling=2^-10  DoSatur=off
  Sum : Sum  Inputs=|+-
  Sum1 : Sum  Inputs=|++
  x_slow : Outport
  wires:
  Gain1/1 -> Saturation Dynamic2/3
  ratedown/1 -> Gain1/1
  rateup/1 -> Gain/1
  Gain/1 -> Saturation Dynamic2/1
  x0/1 -> Delay/2
  Sum1/1 -> Delay/1, x_slow/1
  Saturation Dynamic2/1 -> Sum1/1
  Sum/1 -> Saturation Dynamic2/2
  Delay/1 -> Sum/2, Sum1/2
  x/1 -> Sum/1

== system ControLibrary/HSS/MANAGEMENT/RateLimit/ratelimit1 ==
  rateup : Inport
  x : Inport  Port=2
  ratedown : Inport  Port=3
  x0 : Inport  Port=4
  Delay : Delay  DelayLength=1  InitialConditionSource=Input port  SampleTime=Ts
      settings: InputPortMap=u0,p4
  Gain : Gain  Gain=Ts
  Gain1 : Gain  Gain=-Ts
  Saturation Dynamic2 : simulink/Discontinuities/Saturation Dynamic  OutMin=[]  OutMax=[]  OutDataTypeStr=Inherit: Same as second input  OutDataType=fixdt(1, 16)  OutScaling=2^-10  DoSatur=off
  Sum : Sum  Inputs=|+-
  Sum1 : Sum  Inputs=|++
  x_slow : Outport
  wires:
  Gain1/1 -> Saturation Dynamic2/3
  ratedown/1 -> Gain1/1
  rateup/1 -> Gain/1
  Gain/1 -> Saturation Dynamic2/1
  x0/1 -> Delay/2
  Sum1/1 -> Delay/1, x_slow/1
  Saturation Dynamic2/1 -> Sum1/1
  Sum/1 -> Saturation Dynamic2/2
  Delay/1 -> Sum/2, Sum1/2
  x/1 -> Sum/1

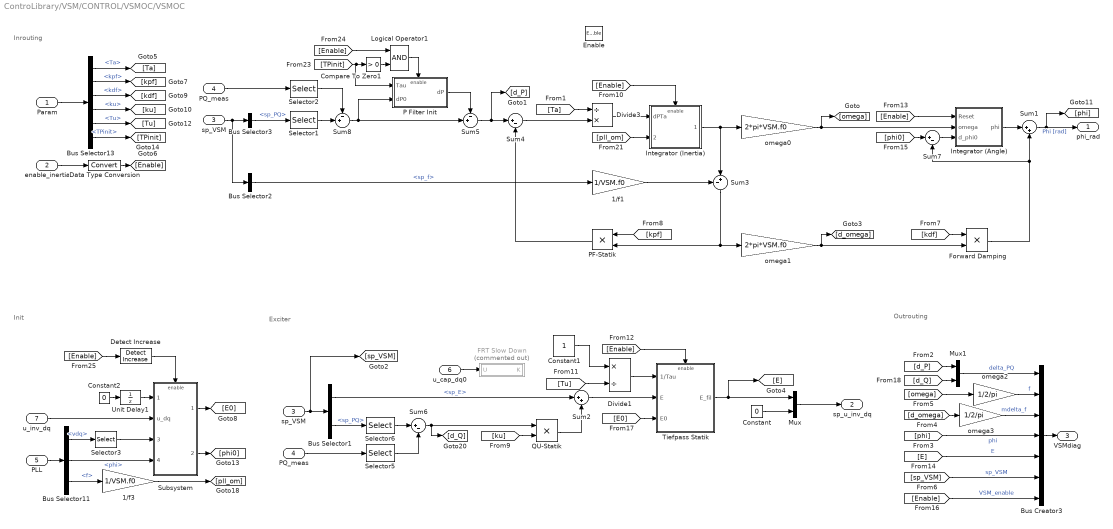
== system ControLibrary/VSM/CONTROL/VSMOC/VSMOC ==
  note: Outrouting
  note: Init
  note: Exciter
  note: Inrouting
  Param : Inport
  enable_inertia : Inport  Port=2
  sp_VSM : Inport  Port=3
  PQ_meas : Inport  Port=4
  PLL : Inport  Port=5
  u_cap_dq0 : Inport  Port=6
  u_inv_dq : Inport  Port=7
  Enable : EnablePort  StatesWhenEnabling=reset
  1/f1 : Gain  Gain=1/VSM.f0
  1/f3 : Gain  Gain=1/VSM.f0
  Bus Creator3 : BusCreator  Inputs=7
  Bus Selector1 : BusSelector  OutputSignals=sp_E,sp_PQ
  Bus Selector11 : BusSelector  OutputSignals=vdq,phi,f
  Bus Selector13 : BusSelector  OutputSignals=Ta,kpf,kdf,ku,Tu,TPinit
  Bus Selector2 : BusSelector  OutputSignals=sp_f
  Bus Selector3 : BusSelector  OutputSignals=sp_PQ
  Compare To Zero1 : simulink/Logic and Bit Operations/Compare To Zero  relop=>  OutDataTypeStr=boolean
  Constant : Constant  Value=0
  Constant1 : Constant
  Constant2 : Constant  Value=0  SampleTime=ControlSampleTime
  Data Type Conversion : DataTypeConversion
  Detect Increase : simulink/Logic and Bit Operations/Detect Increase  vinit=0.0  InputProcessing=Inherited  OutDataTypeStr=boolean
  Divide1 : Product  Inputs=*/
  Divide3 : Product  Inputs=/*
  FRT Slow Down : Subsystem  Commented=on
  Forward Damping : Product  Inputs=**
  Integrator (Angle) : Subsystem
  Integrator (Inertia) : Subsystem
  Logical Operator1 : Logic  AllPortsSameDT=off  OutDataTypeStr=boolean
  Mux : Mux  Inputs=2
  Mux1 : Mux  Inputs=2
  P Filter Init : Subsystem
  PF-Statik : Product  Inputs=**
  "PQ_meas " : InportShadow  Port=4
  QU-Statik : Product  Inputs=**
  Selector1 : Selector  InputPortWidth=2  IndexOptions=Index vector (dialog)  Indices=1  OutputSizes=1
  Selector2 : Selector  InputPortWidth=2  IndexOptions=Index vector (dialog)  Indices=1  OutputSizes=1
  Selector3 : Selector  InputPortWidth=3  IndexOptions=Index vector (dialog)  Indices=[1 2]  OutputSizes=1
  Selector5 : Selector  InputPortWidth=2  IndexOptions=Index vector (dialog)  Indices=2  OutputSizes=1
  Selector6 : Selector  InputPortWidth=2  IndexOptions=Index vector (dialog)  Indices=2  OutputSizes=1
  Subsystem : Subsystem
  Sum1 : Sum  Inputs=|++
  Sum2 : Sum  Inputs=|++
  Sum3 : Sum  Inputs=-+|
  Sum4 : Sum  Inputs=|+-
  Sum5 : Sum  Inputs=-+|
  Sum6 : Sum  Inputs=|+-
  Sum7 : Sum  Inputs=|+-
  Sum8 : Sum  Inputs=-+|
  Tiefpass Statik : Subsystem
  Unit Delay1 : UnitDelay  InitialCondition=1  SampleTime=ControlSampleTime
  omega0 : Gain  Gain=2*pi*VSM.f0
  omega1 : Gain  Gain=2*pi*VSM.f0
  omega2 : Gain  Gain=1/2/pi
  omega3 : Gain  Gain=1/2/pi
  "sp_VSM " : InportShadow  Port=3
  phi_rad : Outport
  sp_u_inv_dq : Outport  Port=2  InitialOutput=[1 0]
  VSMdiag : Outport  Port=3
  wires:
  Constant1/1 -> Divide1/1
  u_cap_dq0/1 -> FRT Slow Down/1(U)
  [Tu] -> Divide1/2
  Divide1/1 -> Tiefpass Statik/1(1/Tau)
  [E0] -> Tiefpass Statik/3(E0)
  enable_inertia/1 -> Data Type Conversion/1
  [phi] -> Bus Creator3/4  "phi"
  Bus Selector1/1 -> Sum2/1  "<sp_E>"
  QU-Statik/1 -> Sum2/2
  Tiefpass Statik/1(E_fil) -> Mux/1, [E]
  Bus Selector13/6 -> [TPinit]  "<TPinit>"
  [E] -> Bus Creator3/5  "E"
  [ku] -> QU-Statik/2
  Sum2/1 -> Tiefpass Statik/2(E)
  [Enable] -> Integrator (Angle)/1(Reset)
  Data Type Conversion/1 -> [Enable]
  Unit Delay1/1 -> Subsystem/1(first_run)
  Constant2/1 -> Unit Delay1/1
  u_inv_dq/1 -> Subsystem/2(u_dq)
  [Enable] -> Detect Increase/1
  Param/1 -> Bus Selector13/1
  Bus Selector13/1 -> [Ta]  "<Ta>"
  Bus Selector13/2 -> [kpf]  "<kpf>"
  Bus Selector13/3 -> [kdf]  "<kdf>"
  Bus Selector13/4 -> [ku]  "<ku>"
  Bus Selector13/5 -> [Tu]  "<Tu>"
  [Enable] -> Logical Operator1/1
  Logical Operator1/1 -> P Filter Init/Enable
  Compare To Zero1/1 -> Logical Operator1/2
  P Filter Init/1(dP) -> Sum5/1
  [TPinit] -> Compare To Zero1/1, P Filter Init/1(Tau)
  Sum8/1 -> P Filter Init/2(dP0), Sum5/2
  Sum5/1 -> [d_P], Sum4/1
  Selector1/1 -> Sum8/2
  Detect Increase/1 -> Subsystem/Enable
  Subsystem/2(u_ang) -> [phi0]
  Subsystem/1(u_abs) -> [E0]
  Constant/1 -> Mux/2
  Mux/1 -> sp_u_inv_dq/1
  [pll_om] -> Integrator (Inertia)/2(omega0 [pu])
  Divide3/1 -> Integrator (Inertia)/1(dPTa)
  Integrator (Inertia)/1(omega [pu]) -> Sum3/2, omega0/1
  Bus Selector11/1 -> Selector3/1  "<vdq>"
  PQ_meas/1 -> Selector2/1
  [sp_VSM] -> Bus Creator3/6  "sp_VSM"
  omega3/1 -> Bus Creator3/3  "mdelta_f"
  omega2/1 -> Bus Creator3/2  "f"
  [d_omega] -> omega3/1
  omega1/1 -> [d_omega], Forward Damping/2
  [omega] -> omega2/1
  Bus Creator3/1 -> VSMdiag/1
  PLL/1 -> Bus Selector11/1
  Bus Selector2/1 -> 1/f1/1  "<sp_f>"
  Bus Selector3/1 -> Selector1/1  "<sp_PQ>"
  omega0/1 -> Integrator (Angle)/2(omega), [omega]
  Sum3/1 -> omega1/1, PF-Statik/2
  Sum4/1 -> Divide3/2
  PF-Statik/1 -> Sum4/2
  Sum1/1 -> phi_rad/1, [phi]  "Phi [rad]"
  [Ta] -> Divide3/1
  [Enable] -> Bus Creator3/7  "VSM_enable"
  Selector3/1 -> Subsystem/3(u_dq_pll)
  Integrator (Angle)/1(phi) -> Sum1/1
  Bus Selector11/3 -> 1/f3/1  "<f>"
  1/f3/1 -> [pll_om]
  [kdf] -> Forward Damping/1
  [kpf] -> PF-Statik/1
  sp_VSM/1 -> Bus Selector3/1, Bus Selector2/1
  "PQ_meas "/1 -> Selector5/1
  Bus Selector1/2 -> Selector6/1  "<sp_PQ>"
  "sp_VSM "/1 -> Bus Selector1/1, [sp_VSM]
  Sum6/1 -> [d_Q], QU-Statik/1
  Selector2/1 -> Sum8/1
  Mux1/1 -> Bus Creator3/1  "delta_PQ"
  [d_P] -> Mux1/1
  [d_Q] -> Mux1/2
  1/f1/1 -> Sum3/1
  Selector6/1 -> Sum6/1
  Selector5/1 -> Sum6/2
  Bus Selector11/2 -> Subsystem/4(phi_pll)  "<phi>"
  Forward Damping/1 -> Sum7/2, Sum1/2
  Sum7/1 -> Integrator (Angle)/3(d_phi0)
  [phi0] -> Sum7/1
  [Enable] -> Integrator (Inertia)/Enable
  [Enable] -> Tiefpass Statik/Enable

== system ControLibrary/VSM/CONTROL/i_dq_ctrl/PI ==
  di : Inport
  u0 : Inport  Port=2
  Enable : EnablePort  StatesWhenEnabling=reset
  Gain4 : Gain  Gain=Ki
  Gain5 : Gain  Gain=Kp
  Integrator (inertia) : DiscreteIntegrator  gainval=1  InitialConditionSource=external  InitialCondition=1  InitialConditionSetting=State (most efficient)  SampleTime=ControlSampleTime  ICPrevOutput=DiscIntNeverNeededParam  ICPrevScaledInput=DiscIntNeverNeededParam
  Sum2 : Sum  Inputs=++|
  u : Outport
  wires:
  Gain4/1 -> Integrator (inertia)/1
  Gain5/1 -> Sum2/1
  Integrator (inertia)/1 -> Sum2/2
  di/1 -> Gain5/1, Gain4/1
  Sum2/1 -> u/1
  u0/1 -> Integrator (inertia)/2

== system ControLibrary/VSM/MANAGEMENT/sp_VSM/E(PQ) ==
  E : Inport
  cmd : Inport  Port=2
  sp_PQ : Inport  Port=3
  Abs : Abs
  Add : Sum
  Add1 : Sum
  Add2 : Sum
  Bus Selector : BusSelector  OutputSignals=Param.VC.R1,Param.VC.R1t,Param.VC.L1,Param.VC.L1t
  Bus Selector1 : BusSelector  OutputSignals=Param.VSM.sp_E_comp
  Demux : Demux  Outputs=2
  Divide : Product  Inputs=/*
  Product : Product
  Real-Imag to Complex : RealImagToComplex
  Real-Imag to Complex1 : RealImagToComplex
  Switch : Switch  Criteria=u2 ~= 0
  "cmd " : InportShadow  Port=2
  sp_E : Outport
  wires:
  Bus Selector1/1 -> Switch/2  "<sp_E_comp>"
  "cmd "/1 -> Bus Selector1/1
  Switch/1 -> sp_E/1
  cmd/1 -> Bus Selector/1
  Bus Selector/1 -> Add/1  "<R1>"
  Bus Selector/2 -> Add/2  "<R1t>"
  Bus Selector/3 -> Add1/1  "<L1>"
  Bus Selector/4 -> Add1/2  "<L1t>"
  Add/1 -> Real-Imag to Complex/1
  Add1/1 -> Real-Imag to Complex/2
  E/1 -> Divide/1, Add2/1, Switch/3
  sp_PQ/1 -> Demux/1
  Demux/1 -> Real-Imag to Complex1/1
  Demux/2 -> Real-Imag to Complex1/2
  Real-Imag to Complex1/1 -> Divide/2
  Divide/1 -> Product/1  "current"
  Real-Imag to Complex/1 -> Product/2  "impedance"
  Product/1 -> Add2/2  "voltage"
  Abs/1 -> Switch/1
  Add2/1 -> Abs/1

== system ControLibrary/VSM/MANAGEMENT/sp_VSM/PQ(U) Limit ==
  sp_PQ : Inport
  enable : Inport  Port=2
  u_out : Inport  Port=3
  Demux : Demux  Outputs=2
  Demux1 : Demux  Outputs=2
  Math Function : Math  Operator=hypot  SaturateOnIntegerOverflow=on
  MinMax : MinMax  Inputs=2
  Mux : Mux  Inputs=2
  Selector2 : Selector  InputPortWidth=3  IndexOptions=Index vector (dialog)  Indices=[1 2]  OutputSizes=1
  Switch : Switch  Criteria=u2 ~= 0
  sp_PQ_limit : Outport
  wires:
  enable/1 -> Switch/2
  Switch/1 -> sp_PQ_limit/1
  Mux/1 -> Switch/1
  MinMax/1 -> Mux/1
  Demux1/1 -> MinMax/2
  Demux1/2 -> Mux/2
  sp_PQ/1 -> Demux1/1, Switch/3
  u_out/1 -> Selector2/1
  Math Function/1 -> MinMax/1
  Demux/2 -> Math Function/2
  Demux/1 -> Math Function/1
  Selector2/1 -> Demux/1

== system ControLibrary/VSM/MANAGEMENT/sp_VSM/RateLimit ==
  PQ : Inport
  Enable : EnablePort
  Compare To Zero : simulink/Logic and Bit Operations/Compare To Zero  relop=>  OutDataTypeStr=boolean
  Constant1 : Constant  Value=Mgn.PQSpRateUp  SampleTime=ControlSampleTime
  Constant2 : Constant  Value=Mgn.PQSpRateDown  SampleTime=ControlSampleTime
  Constant6 : Constant  Value=Mgn.PQSpRateDown  SampleTime=ControlSampleTime
  Constant7 : Constant  Value=Mgn.PQSpRateUp  SampleTime=ControlSampleTime
  Constant8 : Constant  Value=[0 0]  SampleTime=ControlSampleTime
  Logical Operator : Logic  Inputs=1  AllPortsSameDT=off  OutDataTypeStr=boolean
  Mux : Mux  Inputs=2
  Switch : Switch  Criteria=u2 > Threshold
  ratelimitspPQ : Subsystem  mask{Ts=ControlSampleTime}
      mask DialogControl ParameterGroupVar Prompt: Rate Limiter
  PQslow : Outport
  wires:
  PQ/1 -> Switch/3, ratelimitspPQ/2(x)
  ratelimitspPQ/1(x_slow) -> Switch/1
  Constant8/1 -> ratelimitspPQ/4(x0)
  Constant6/1 -> ratelimitspPQ/3(ratedown)
  Switch/1 -> PQslow/1  "sp_PQ"
  Constant7/1 -> ratelimitspPQ/1(rateup)
  Compare To Zero/1 -> Logical Operator/1
  Constant1/1 -> Mux/1
  Constant2/1 -> Mux/2
  Mux/1 -> Compare To Zero/1
  Logical Operator/1 -> Switch/2

== system ControLibrary/VSMCC/CONTROL/VSMOC/Integrator (Angle) ==
  Reset : Inport
  omega : Inport  Port=2
  phi0 : Inport  Port=3
  Angle Integrator Reset[SI] : FriedrichLibrary/Discrete Stuff/Angle Integrator Reset[SI]  Ts=ControlSampleTime
  Delay : Delay  DelayLength=1  InitialConditionSource=Input port
      settings: InputPortMap=u0,p4
  Gain3 : Gain  Gain=-ControlSampleTime
  Sum1 : Sum  Inputs=|++
  Sum9 : Sum  Inputs=|+-
  phi : Outport
  wires:
  Gain3/1 -> Delay/2, Sum9/2
  omega/1 -> Gain3/1, Angle Integrator Reset[SI]/2
  Angle Integrator Reset[SI]/1 -> Delay/1, phi/1  "Phi [rad]"
  Reset/1 -> Angle Integrator Reset[SI]/1
  Sum9/1 -> Sum1/1
  Sum1/1 -> Angle Integrator Reset[SI]/3
  phi0/1 -> Sum9/1
  Delay/1 -> Sum1/2

== system ControLibrary/VSMCC/CONTROL/VSMOC/Integrator (Inertia) ==
  dPTa : Inport
  omega_0 : Inport  Port=2
  Enable : EnablePort
  Integrator (inertia) : DiscreteIntegrator  gainval=1  InitialConditionSource=external  InitialCondition=1  InitialConditionSetting=State (most efficient)  SampleTime=ControlSampleTime  ICPrevOutput=DiscIntNeverNeededParam  ICPrevScaledInput=DiscIntNeverNeededParam
  omega : Outport
  wires:
  omega_0/1 -> Integrator (inertia)/2
  Integrator (inertia)/1 -> omega/1  "Omega [pu]"
  dPTa/1 -> Integrator (inertia)/1

== system ControLibrary/VSMCC/CONTROL/VSMOC/P Filter Init ==
  Tau : Inport
  dP0 : Inport  Port=2
  Enable : EnablePort  StatesWhenEnabling=reset
  Divide4 : Product  Inputs=*/
  Gain : Gain  Gain=-1
  Integrator1 : DiscreteIntegrator  gainval=1  InitialConditionSource=external  InitialConditionSetting=State (most efficient)  SampleTime=ControlSampleTime  ICPrevOutput=DiscIntNeverNeededParam  ICPrevScaledInput=DiscIntNeverNeededParam
  dP : Outport
  wires:
  dP0/1 -> Integrator1/2
  Gain/1 -> Divide4/1
  Divide4/1 -> Integrator1/1
  Tau/1 -> Divide4/2
  Integrator1/1 -> dP/1, Gain/1

== system ControLibrary/VSMCC/CONTROL/VSMOC/Subsystem ==
  first_run : Inport
  u_dq : Inport  Port=2
  u_dq_pll : Inport  Port=3
  phi_pll : Inport  Port=4
  Enable : EnablePort
  Complex to Magnitude-Angle : ComplexToMagnitudeAngle
  Demux : Demux  Outputs=2
  Real-Imag to Complex : RealImagToComplex
  Switch : Switch  Criteria=u2 > Threshold
  Switch1 : Switch  Criteria=u2 > Threshold
  "first_run " : InportShadow
  u_abs : Outport  InitialOutput=1
  u_ang : Outport  Port=2  InitialOutput=0
  wires:
  Switch/1 -> u_ang/1
  phi_pll/1 -> Switch/1
  Complex to Magnitude-Angle/2 -> Switch/3
  Real-Imag to Complex/1 -> Complex to Magnitude-Angle/1
  Demux/1 -> Real-Imag to Complex/1
  Demux/2 -> Real-Imag to Complex/2
  Complex to Magnitude-Angle/1 -> u_abs/1
  Switch1/1 -> Demux/1
  first_run/1 -> Switch1/2
  u_dq/1 -> Switch1/3
  u_dq_pll/1 -> Switch1/1
  "first_run "/1 -> Switch/2

== system ControLibrary/VSMCC/CONTROL/VSMOC/Tiefpass Statik ==
  Tau : Inport
  spE : Inport  Port=2
  dEQ : Inport  Port=3
  E0 : Inport  Port=4
  Enable : EnablePort  StatesWhenEnabling=reset
  Divide1 : Product  Inputs=/*
  Integrator : DiscreteIntegrator  gainval=1  InitialConditionSource=external  InitialCondition=0.9  InitialConditionSetting=State (most efficient)  SampleTime=ControlSampleTime  ICPrevOutput=DiscIntNeverNeededParam  ICPrevScaledInput=DiscIntNeverNeededParam
  Sum1 : Sum  Inputs=++-
  Sum6 : Sum  Inputs=|+-
  E : Outport
  wires:
  dEQ/1 -> Sum1/1
  Sum6/1 -> Sum1/2
  spE/1 -> Sum6/1
  E0/1 -> Integrator/2
  Sum1/1 -> Divide1/2
  Divide1/1 -> Integrator/1
  Integrator/1 -> E/1, Sum6/2  "E [pu]"
  Tau/1 -> Divide1/1

== system ControLibrary/VSMCC/CONTROL/active_damping/VTFF - HighPass1 ==
  u : Inport
  Enable : EnablePort  StatesWhenEnabling=reset
  Constant : Constant  Value=Tlag
  Gain1 : Gain  Gain=Gain
  Gain2 : Gain  Gain=OmLag
  Gain3 : Gain  Gain=Tlead
  Gain4 : Gain  Gain=Gain
  Gain5 : Gain  Gain=OmLag
  Sum : Sum  Inputs=|+-
  Sum1 : Sum  Inputs=++|
  Switch : Switch  Criteria=u2 > Threshold
  init : Constant  Value=0
  integrator : ctrl_basic/integrator  SystemSampleTime=-1
  "u " : InportShadow
  x : Outport
  wires:
  u/1 -> Gain4/1
  Sum/1 -> integrator/1
  Sum1/1 -> Switch/1, Gain5/1
  Gain5/1 -> Sum/2
  integrator/1 -> Sum1/2
  Gain3/1 -> Sum1/1
  init/1 -> integrator/2
  Constant/1 -> Switch/2
  Switch/1 -> x/1
  Gain4/1 -> Gain2/1
  Gain2/1 -> Sum/1, Gain3/1
  "u "/1 -> Gain1/1
  Gain1/1 -> Switch/3

== system ControLibrary/VSMCC/CONTROL/active_damping/VTFF - HighPass2 ==
  u : Inport
  Enable : EnablePort  StatesWhenEnabling=reset
  Constant : Constant  Value=Tlag
  Gain1 : Gain  Gain=Gain
  Gain2 : Gain  Gain=OmLag
  Gain3 : Gain  Gain=Tlead
  Gain4 : Gain  Gain=Gain
  Gain5 : Gain  Gain=OmLag
  Sum : Sum  Inputs=|+-
  Sum1 : Sum  Inputs=++|
  Switch : Switch  Criteria=u2 > Threshold
  init : Constant  Value=0
  integrator : ctrl_basic/integrator  SystemSampleTime=-1
  "u " : InportShadow
  x : Outport
  wires:
  Gain1/1 -> Switch/3
  "u "/1 -> Gain1/1
  Gain2/1 -> Sum/1, Gain3/1
  Gain4/1 -> Gain2/1
  Switch/1 -> x/1
  Constant/1 -> Switch/2
  init/1 -> integrator/2
  Gain3/1 -> Sum1/1
  integrator/1 -> Sum1/2
  Gain5/1 -> Sum/2
  Sum1/1 -> Gain5/1, Switch/1
  Sum/1 -> integrator/1
  u/1 -> Gain4/1

== system ControLibrary/VSMCC/CONTROL/i_dq_ctrl/PI ==
  di : Inport
  u0 : Inport  Port=2
  Enable : EnablePort  StatesWhenEnabling=reset
  Gain4 : Gain  Gain=Ki
  Gain5 : Gain  Gain=Kp
  Integrator (inertia) : DiscreteIntegrator  gainval=1  InitialConditionSource=external  InitialCondition=1  InitialConditionSetting=State (most efficient)  SampleTime=ControlSampleTime  ICPrevOutput=DiscIntNeverNeededParam  ICPrevScaledInput=DiscIntNeverNeededParam
  Sum2 : Sum  Inputs=++|
  u : Outport
  wires:
  Gain4/1 -> Integrator (inertia)/1
  Gain5/1 -> Sum2/1
  Integrator (inertia)/1 -> Sum2/2
  di/1 -> Gain5/1, Gain4/1
  Sum2/1 -> u/1
  u0/1 -> Integrator (inertia)/2

== system ControLibrary/VSM/CONTROL/VSMOC/VSMOC/FRT Slow Down ==
  U : Inport
  Bias : Bias  Bias=0.2
  Complex to Magnitude-Angle : ComplexToMagnitudeAngle
  Demux : Demux  Outputs=2
  Real-Imag to Complex : RealImagToComplex
  Saturation : Saturate  UpperLimit=1  LowerLimit=0
  Terminator : Terminator
  Unit Delay4 : UnitDelay  SampleTime=ControlSampleTime
  K : Outport
  wires:
  Unit Delay4/1 -> Demux/1
  Saturation/1 -> K/1
  Bias/1 -> Saturation/1
  Complex to Magnitude-Angle/2 -> Terminator/1
  U/1 -> Unit Delay4/1
  Real-Imag to Complex/1 -> Complex to Magnitude-Angle/1
  Demux/1 -> Real-Imag to Complex/1
  Demux/2 -> Real-Imag to Complex/2
  Complex to Magnitude-Angle/1 -> Bias/1

== system ControLibrary/VSM/CONTROL/VSMOC/VSMOC/Integrator (Angle) ==
  Reset : Inport
  omega : Inport  Port=2
  d_phi0 : Inport  Port=3
  Angle Integrator Reset[SI] : FriedrichLibrary/Discrete Stuff/Angle Integrator Reset[SI]  Ts=ControlSampleTime
  Delay : Delay  DelayLength=1  InitialConditionSource=Input port
      settings: InputPortMap=u0,p4
  Gain3 : Gain  Gain=-1*ControlSampleTime
  Sum1 : Sum  Inputs=|++
  Sum9 : Sum  Inputs=|+-
  phi : Outport
  wires:
  Delay/1 -> Sum1/2
  d_phi0/1 -> Sum9/1
  Sum1/1 -> Angle Integrator Reset[SI]/3
  Sum9/1 -> Sum1/1
  Reset/1 -> Angle Integrator Reset[SI]/1
  Angle Integrator Reset[SI]/1 -> phi/1, Delay/1  "Phi [rad]"
  omega/1 -> Angle Integrator Reset[SI]/2, Gain3/1
  Gain3/1 -> Sum9/2, Delay/2
